simulink model "PMSMOpenLoopControl"  (R2022a)
settings: Solver=ode1  StartTime=0.0  StopTime=10  FixedStep=1e-5  RelTol=1e-3
values from neighbouring files (symbols this model uses):
  A = [0 -Lq  ; Ld 0 ]    [PMSMParameters.m]
  C0 = 3.53*10.^-1    (= 0.353)    [PMSMParameters.m]
  F = 1.57*10.^-3    (= 0.00157)    [PMSMParameters.m]
  J = 5.21*10.^-3    (= 0.00521)    [PMSMParameters.m]
  Kim = J*((wnm).^2)/Kpm    [PMSMParameters.m]
  Kpm = 2*wnm*J*ceff-F    (= 0.25893)    [PMSMParameters.m]
  L = [Ld 0 ; 0 Lq ]    [PMSMParameters.m]
  Lq = 0.23    [PMSMParameters.m]
  P = 2    [PMSMParameters.m]
  pf = 1.12    [PMSMParameters.m]
  phif = [0 ; pf]    [PMSMParameters.m]
  R = [Rs 0; 0 Rs ]    [PMSMParameters.m]
  Rs = 27.9    [PMSMParameters.m]
settings Model: Creator=ZinouAb  LastModifiedBy=ZinouAb
settings ModelReferenceCC: EnableRefExpFcnMdlSchedulingChecks=off
settings RTWCC: Description=Generic Real-Time Target

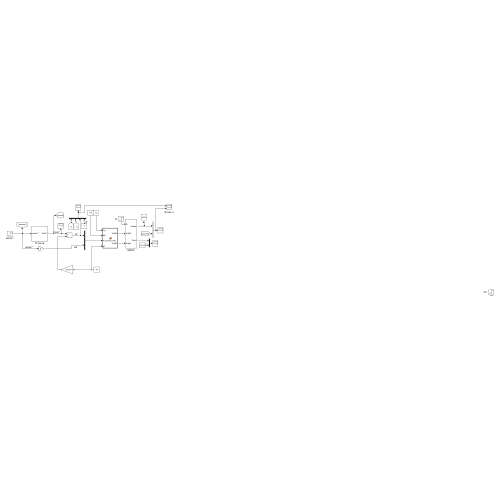
[thumbnail: Simulink's stored preview of the top-level diagram]
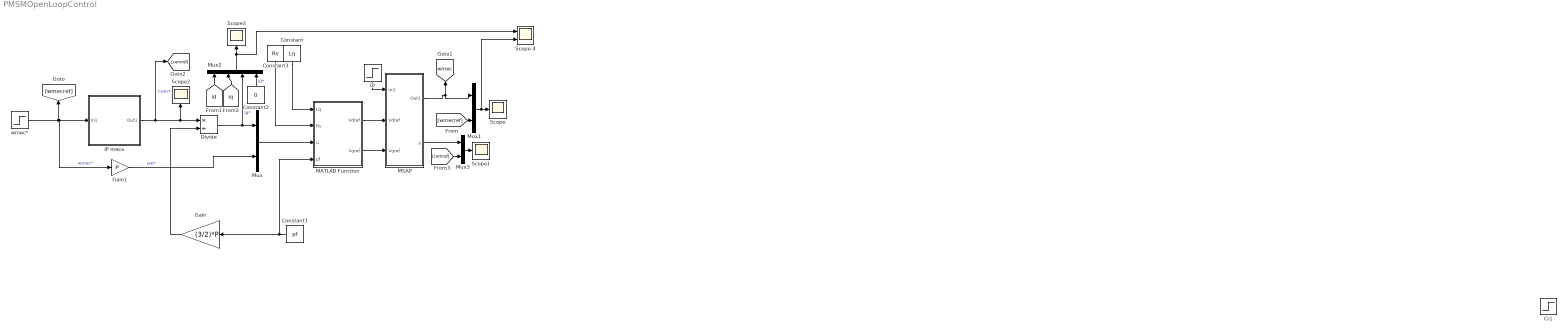
== system PMSMOpenLoopControl ==
  Constant : Constant  Value=Lq
  Constant1 : Constant  Value=pf
  Constant2 : Constant  Value=0
  Constant3 : Constant  Value=Rs
  Cr : Step  Time=6  Before=0.5  After=1+C0  SampleTime=0
  Cr1 : Step  Time=2  Before=0.5  After=5  SampleTime=0
  Divide : Product  Inputs=*/
  Gain : Gain  Gain=(3/2)*P
  Gain1 : Gain  Gain=P
  IP meca : Subsystem
  MATLAB Function : MATLAB Function  TreatAsAtomicUnit=on
  MSAP : Subsystem
  Mux : Mux  Inputs=2
  Mux1 : Mux  Inputs=2
  Mux2 : Mux
  Mux3 : Mux  Inputs=2
  Scope{,1..3} (4 alike) : Scope
  Scope 4 : Scope  NumInputPorts=2
  wmec* : Step  Time=4  After=157  SampleTime=0
  tag scope: wmec=global
  wires:
  Gain1/1 -> Mux/2  "we*"
  [wmecref] -> Mux1/2
  Divide/1 -> Mux/1, Mux2/3  "Iq*"
  Constant1/1 -> Gain/1, MATLAB Function/4(pf)
  [id] -> Mux2/1
  Cr/1 -> MSAP/1(In3)
  Gain/1 -> Divide/2
  IP meca/1(Out1) -> [cemref], Divide/1, Scope2/1  "Cem*"
  Mux2/1 -> Scope 4/1, Scope3/1
  MSAP/2(y) -> Mux3/1
  MATLAB Function/2(Vqref) -> MSAP/3(Vqref)
  Constant/1 -> MATLAB Function/1(Lq)
  MSAP/1(Out1) -> [wmec], Mux1/1
  Mux/1 -> MATLAB Function/3(u)
  wmec*/1 -> IP meca/1(In1), Gain1/1, [wmecref]  "wmec*"
  Constant3/1 -> MATLAB Function/2(Rs)
  [iq] -> Mux2/2
  MATLAB Function/1(Vdref) -> MSAP/2(Vdref)
  [cemref] -> Mux3/2
  Mux3/1 -> Scope1/1
  Constant2/1 -> Mux2/4  "id*"
  Mux1/1 -> Scope 4/2, Scope/1

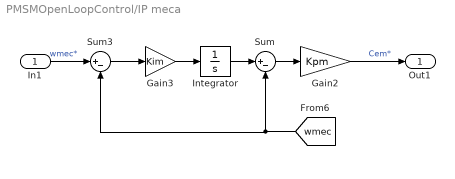
== system PMSMOpenLoopControl/IP meca ==
  In1 : Inport
  Gain2 : Gain  Gain=Kpm
  Gain3 : Gain  Gain=Kim
  Integrator : Integrator
  Sum : Sum  Inputs=|+-
  Sum3 : Sum  Inputs=|+-
  Out1 : Outport
  wires:
  Integrator/1 -> Sum/1
  [wmec] -> Sum3/2, Sum/2
  Sum/1 -> Gain2/1
  Gain2/1 -> Out1/1  "Cem*"
  Gain3/1 -> Integrator/1
  Sum3/1 -> Gain3/1
  In1/1 -> Sum3/1  "wmec*"

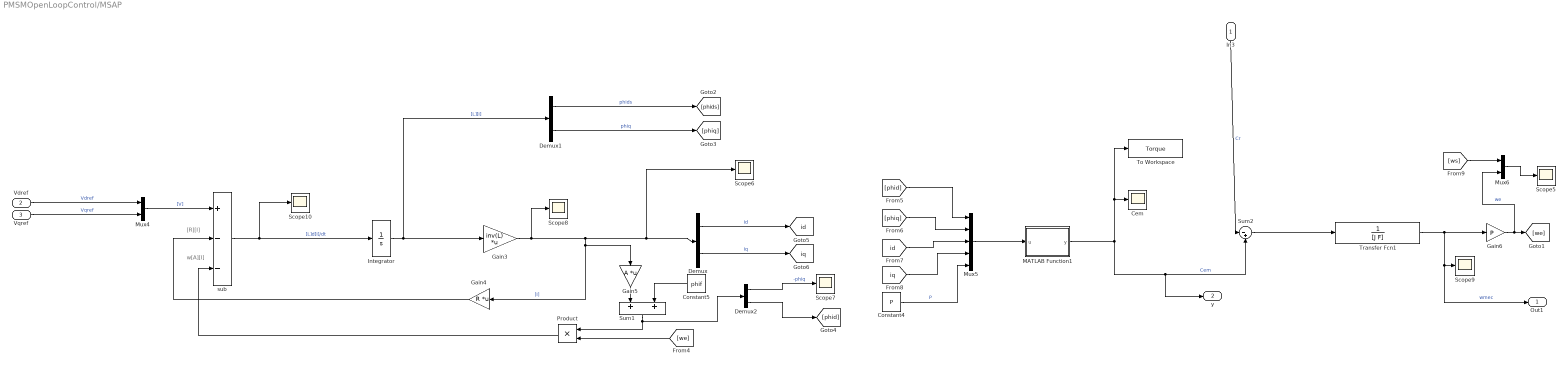
== system PMSMOpenLoopControl/MSAP ==
  note: [R][I]
  note: w[A][I]
  In3 : Inport
  Vdref : Inport  Port=2
  Vqref : Inport  Port=3
  Cem : Scope
  Constant4 : Constant  Value=P
  Constant5 : Constant  Value=phif
  Demux : Demux  Outputs=2
  Demux1 : Demux  Outputs=2
  Demux2 : Demux  Outputs=2
  Gain3 : Gain  Gain=inv(L)  Multiplication=Matrix(K*u)
  Gain4 : Gain  Gain=R  Multiplication=Matrix(K*u)
  Gain5 : Gain  Gain=A  Multiplication=Matrix(K*u)
  Gain6 : Gain  Gain=P
  Integrator : Integrator
  MATLAB Function1 : MATLAB Function  TreatAsAtomicUnit=on
  Mux4 : Mux  Inputs=2
  Mux5 : Mux  Inputs=5
  Mux6 : Mux  Inputs=2
  Product : Product
  Scope{5..10} (6 alike) : Scope
  Sum1 : Sum
  Sum2 : Sum  Inputs=|-+
  To Workspace : ToWorkspace  VariableName=Torque  SaveFormat=Timeseries  SampleTime=-1
  Transfer Fcn1 : TransferFcn  Denominator=[J F]
  sub : Sum  Inputs=+--
  Out1 : Outport
  y : Outport  Port=2
  tag scope: id=global, iq=global
  wires:
  sub/1 -> Scope10/1, Integrator/1  "[L]d[I]/dt"
  MATLAB Function1/1(y) -> To Workspace/1, Cem/1, y/1, Sum2/2  "Cem"
  Product/1 -> sub/3
  Sum2/1 -> Transfer Fcn1/1
  Transfer Fcn1/1 -> Out1/1, Scope9/1, Gain6/1  "wmec"
  Vdref/1 -> Mux4/1  "Vdref"
  Gain4/1 -> sub/2
  Gain6/1 -> Mux6/2, [we]  "we"
  Demux/2 -> [iq]  "Iq"
  Sum1/1 -> Product/1, Demux2/1
  Demux1/2 -> [phiq]  "phiq"
  Integrator/1 -> Gain3/1, Demux1/1  "[L][I]"
  Mux6/1 -> Scope5/1
  Constant4/1 -> Mux5/5  "P"
  Demux/1 -> [id]  "Id"
  [we] -> Product/2
  Gain5/1 -> Sum1/1
  Gain3/1 -> Gain4/1, Gain5/1, Scope6/1, Demux/1, Scope8/1  "[I]"
  Vqref/1 -> Mux4/2  "Vqref"
  Mux5/1 -> MATLAB Function1/1(u)
  In3/1 -> Sum2/1  "Cr"
  Constant5/1 -> Sum1/2
  [id] -> Mux5/3
  [iq] -> Mux5/4
  Demux2/2 -> [phid]
  Demux2/1 -> Scope7/1  "-phiq"
  Mux4/1 -> sub/1  "[V]"
  Demux1/1 -> [phids]  "phids"
  [phid] -> Mux5/1
  [phiq] -> Mux5/2
  [ws] -> Mux6/1

== matlab function PMSMOpenLoopControl/MATLAB Function ==
  data: Lq input; Rs input; u input; pf input; Vdref output; Vqref output
function [Vdref,Vqref] = Correcteurelec(Lq,Rs,u,pf)
Vdref=-u(2)*Lq*u(1);
Vqref=u(2)*pf+Rs*u(1);

== matlab function PMSMOpenLoopControl/MSAP/MATLAB Function1 ==
  data: u input; y output
function y = CEM(u)

y =(3/2)*u(5)*(u(1)*u(4)-u(2)*u(3));
